simulink library "angleBtw2Vecs_ul"  (R2020a)
settings: Solver=VariableStepAuto  StartTime=0.0  StopTime=10.0  RelTol=1e-3
libraries: vrlib x1
settings Model: Creator=James Reed  LastModifiedBy=John Jr
settings DataIOCC: ReturnWorkspaceOutputs=off
settings DebuggingCC: ArithmeticOperatorsInVariantConditions=warning
settings SFSimCC: CustomCodeUndefinedFunction=UseInterfaceOnly

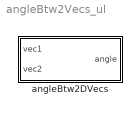
== system angleBtw2Vecs_ul ==
  angleBtw2DVecs : Subsystem

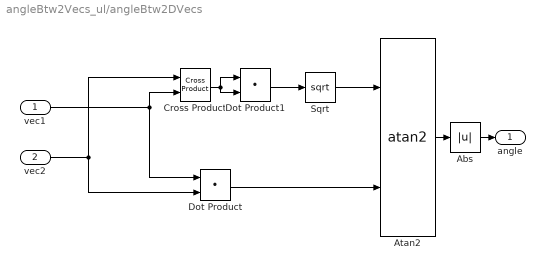
== system angleBtw2Vecs_ul/angleBtw2DVecs ==
  vec1 : Inport
  vec2 : Inport  Port=2
  Abs : Abs
  Atan2 : Trigonometry  Operator=atan2
  Cross Product : vrlib/Utilities/Cross Product
  Dot Product : DotProduct  InputSameDT=on  OutDataTypeStr=Inherit: Inherit via internal rule
  Dot Product1 : DotProduct  InputSameDT=on  OutDataTypeStr=Inherit: Inherit via internal rule
  Sqrt : Sqrt  SaturateOnIntegerOverflow=on
  angle : Outport  VectorParamsAs1DForOutWhenUnconnected=off
  wires:
  Atan2/1 -> Abs/1
  vec1/1 -> Dot Product/1, Cross Product/2
  vec2/1 -> Cross Product/1, Dot Product/2
  Cross Product/1 -> Dot Product1/1, Dot Product1/2
  Dot Product/1 -> Atan2/2
  Abs/1 -> angle/1
  Dot Product1/1 -> Sqrt/1
  Sqrt/1 -> Atan2/1
